simulink model "model"  (R2014a)
settings: Solver=FixedStepDiscrete  StartTime=0.0  StopTime=10.0  RelTol=1e-3
undefined symbols (not defined in the file): ECU565, motohawk_build_version, motohawk_trunc_name, motohawk_vardec_path
libraries: MotoHawk_lib x21
settings Model: MotoHawkModelGUID=11A61F78-2EA3-404C-BC5C-7D2024A9F3B7  MotoHawkModelOpenTime=2016 1 25 15 27 48.637  MotoHawkBuildVersion=007  MotoHawkBuildStats=struct('TotalFLASH',{0},'TotalEEPROM',{0},'TotalRAM',{0},'AppFLASH',{0},'AppEEPROM',{0},'AppRAM',{0},'HeapRAM',{0},'BuildSuccessCount',{7},'BuildErrorCount',{0})  MotoHawkBuildDirectory=H:\EE 5750 Lab\Lab 1\model_Build  MotoHawkBuildInfo=struct('model_name',{'model'},'motohawk_version',{'2014a_sp3.1030'},'motohawk_component_version',{'0.0.8'},'matlab_version',{'8.3.0'},'build_version',{'006'},'module_type',{'ECU565-128'},'layout_type',{'DEV'},'processor_family',{'PPC'},'processor_type',{'MPC565'},'toolchain_vendor',{'gcc-powerpc-eabi'},'toolchain_version',{'4.6.0'},'component',{0},'archive_file',{'PCM128.a'},'enable_build',{1},'fptype',{0},'flash_size',{1048576},'ee_size',{8192},'ram_size',{36864},'decram_size',{4096},'eri_table0_rev',{9},'max_eri_table_size',{65535},'fgnd_base_period_ms',{5},'bgnd_base_period_ms',{50},'build_dir',{'H:\EE 5750 Lab\Lab 1\model_Build'},'dll_name',{'model_006'},'srz_name',{'model_006'},'fgnd_stack_size',{3072},'fgnd_angle_stack_size',{0},'bgnd_stack_size',{2048},'idle_stack_size',{1024},'irq_stack_size',{1536},'heap_size',{4096},'heap_margin',{409},'install_dll_dir',{'C:\ECUFiles\TDBDLL'},'install_srz_dir',{'C:\ECUFiles\Programs'},'app_int_stack_size',{1024},'shutdown_stack_size',{1024},'mingw_dir',{'C:\Program Files (x86)\Woodward\DevelopmentTools\Toolchains\GCC\win32-pe\4_7_0'},'motohawk_dir',{'C:\Program Files (x86)\Woodward\MCS\MotoHawk\2014a_sp3.1030'},'toolchain_dir',{'C:\Program Files (x86)\Woodward\DevelopmentTools\Toolchains\GCC\powerpc-eabi\4_6_0'},'matlab_root',{'C:\Program Files\MATLAB\2014a'},'model_guid',{'11A61F78-2EA3-404C-BC5C-7D2024A9F3B7'},'build_guid',{'7B202DAE-6419-4B4F-BE95-2BA6D031F5CC'},'token_guid',{'FCE0CA5DFB76074BA85E27C6355608D2'})  MotoHawkModelSavedName=model  MotoHawkModelElapsedTime=23442.054  MotoHawkBuildGUID=7B202DAE-6419-4B4F-BE95-2BA6D031F5CC  Creator=lbaruah  LastModifiedBy=lbaruah
settings ConfigSet: Description="This Simulink Configuration Set is preconfigured  for the MotoHawk target \"ECU565-128\"."
settings OptimizationCC: InlineParams=on  InlineInvariantSignals=on  EnhancedBackFolding=on  InitFltsAndDblsToZero=on  NoFixptDivByZeroProtection=on  EfficientFloat2IntCast=on  OptimizeModelRefInitCode=on  LifeSpan=1
settings DebuggingCC: UnderspecifiedInitializationDetection=Classic  SolverPrmCheckMsg=none  InheritedTsInSrcMsg=none  TasksWithSamePriorityMsg=none
settings HardwareCC: ProdLargestAtomicInteger=Integer  ProdLargestAtomicFloat=Float  ProdEndianess=BigEndian  ProdHWDeviceType=Specified
settings ModelReferenceCC: UpdateModelReferenceTargets=AssumeUpToDate  CheckModelReferenceTargetMessage=none  ModelReferenceNumInstancesAllowed=Zero
settings RTWCC: SystemTargetFile=motohawk_ert_rtw.tlc  MakeCommand=motohawk_make_rtw  TemplateMakefile=motohawk_ert_rtw.tmf  Description=MotoHawk(tm) Rapid Prototyping  ProcessScript=motohawk_ert_rtw_make_rtw_hook
settings CodeAppCC: IgnoreCustomStorageClasses=off  MaxIdLength=100  CustomSymbolStrType=$N$R$M  CustomSymbolStrField=$H$N$M  InternalIdentifier=Classic
settings STFCustomTargetCC: ERTMultiwordTypeDef=User defined  ModelReferenceCompliant=off  ConcurrentExecutionCompliant=off  IncludeMdlTerminateFcn=off  CombineOutputUpdateFcns=on  SuppressErrorStatus=on  ERTCustomFileBanners=on  SupportContinuousTime=off  SupportNonInlinedSFcns=off  MATLABClassNameForMDSCustomization=Simulink.SoftwareTarget.ERTCustomization  GRTInterface=off  SystemTargetFile=motohawk_ert_rtw.tlc
settings ERTTargetCC: ERTMultiwordTypeDef=User defined  ERTMultiwordLength=0  GenerateSampleERTMain=off  ModelReferenceCompliant=off  IncludeMdlTerminateFcn=off  GeneratePreprocessorConditionals=Disable all  SuppressErrorStatus=on  ERTCustomFileTemplate=example_file_process.tlc

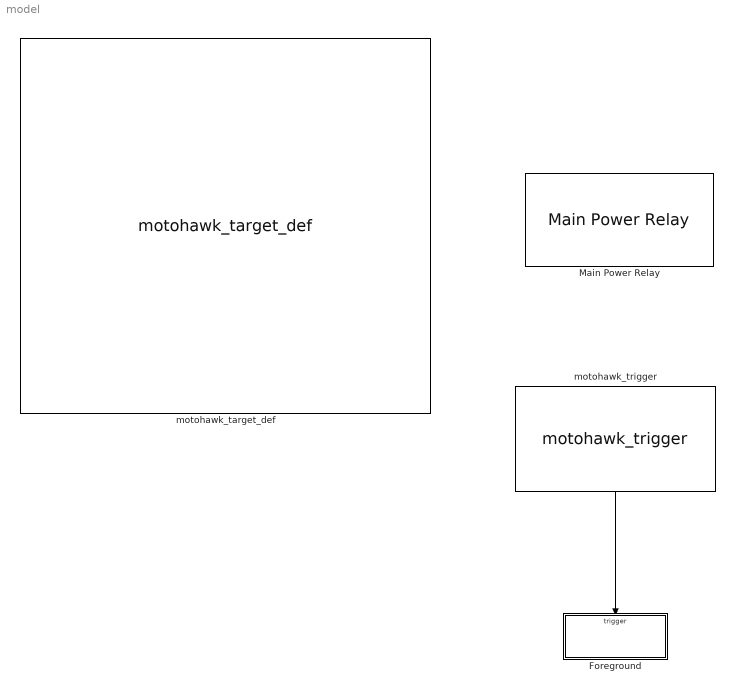
== system model ==
  Foreground : Subsystem  TreatAsAtomicUnit=on
  Main Power Relay : MotoHawk_lib/Extra Development Blocks/Main Power Relay  on_delay_count=2  off_delay_count=5  ecup_threshold=100  group='System | Main Power Relay'
  motohawk_target_def : MotoHawk_lib/motohawk_target_def  Priority=-65535  target=ECU565-128  layout=DEV  fptype=single (32 bits)  fgnd_stack_size=3*1024  fgnd_angle_stack_size=0  bgnd_stack_size=2*1024  idle_stack_size=1024  irq_stack_size=1536  app_int_stack_size=1024  shutdown_stack_size=1024  heap_size=4*1024  show_margins=off  fgnd_stack_margin=(3*1024) * 0.1  fgnd_angle_stack_margin=0  bgnd_stack_margin=(2*1024) * 0.1  idle_stack_margin=(1024) * 0.1  irq_stack_margin=(1536) * 0.1  app_int_stack_margin=(1024) * 0.1  shutdown_stack_margin=(1024) * 0.1  heap_margin=(4*1024) * 0.1  comp_name=bdroot  comp_img='KVASER_CAN_USB.jpg'  comp_security=No Encryption  comp_build_pass='mhbuild'  comp_sim_pass='mhsim'  comp_multi=off  show_filenames=off  dll_name=motohawk_trunc_name(bdroot, ['_' motohawk_build_version], 13)  srz_name=motohawk_trunc_name(bdroot, ['_' motohawk_build_version], 50)  build_dir='.'  comp_dir='.'
  motohawk_trigger : MotoHawk_lib/Trigger Blocks/motohawk_trigger  Tag=Trigger  Priority=0  trig_name=[]  trigger=FGND_RTI_PERIODIC  priority_order=0  inherited=off  run_disabled=off  override_app_monitor=off  target=ECU565_128
  wires:
  motohawk_trigger/1 -> Foreground/Trigger

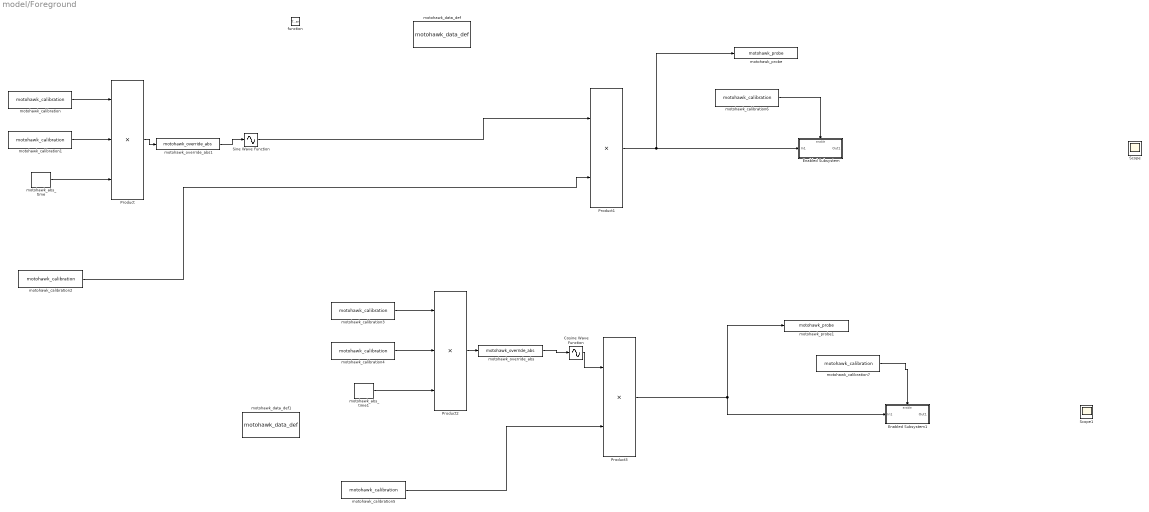
== system model/Foreground ==
  function : TriggerPort  TriggerType=function-call
  Cosine Wave Function : Sin  TimeSource=Use external signal  Phase=pi/2  SampleTime=0
  Enabled Subsystem : Subsystem  TreatAsAtomicUnit=on
  Enabled Subsystem1 : Subsystem  TreatAsAtomicUnit=on
  Product : Product  Inputs=3
  Product1 : Product
  Product2 : Product  Inputs=3
  Product3 : Product
  Scope : Scope
  Scope1 : Scope
  Sine Wave Function : Sin  TimeSource=Use external signal  SampleTime=0
  motohawk_abs_time : MotoHawk_lib/Extra Development Blocks/motohawk_abs_time  mode=Seconds (double)  width=64 bit
  motohawk_abs_time1 : MotoHawk_lib/Extra Development Blocks/motohawk_abs_time  mode=Seconds (double)  width=64 bit
  motohawk_calibration : MotoHawk_lib/Calibration & Probing Blocks/motohawk_calibration  nam='TwoPi'  val=6.28318  storage=Calibration  show_more=off  name_source=Use Parameter  data_type=Inherit from 'Default Value'  read_level=1  write_level=1  ovr_cals=on  view_as=Number  enum_struct={'Disabled', 'Enabled'}  vector_style=Wide Row  use_help_units=off  help=''  units=''  use_header_enum=off  row_header_enum={}  col_header_enum={}  use_min_max=off  min_val=-inf  max_val=inf  use_precision=off  precision=''  gain=1  offset=0  exp=1  use_mototune_group=off  mototune_group=motohawk_vardec_path(gcb)  data_stores=motohawk_sfun_calibration_data_stores
  motohawk_calibration1 : MotoHawk_lib/Calibration & Probing Blocks/motohawk_calibration  nam='f'  val=1  storage=Calibration  show_more=off  name_source=Use Parameter  data_type=Inherit from 'Default Value'  read_level=1  write_level=1  ovr_cals=on  view_as=Number  enum_struct={'Disabled', 'Enabled'}  vector_style=Wide Row  use_help_units=off  help=''  units=''  use_header_enum=off  row_header_enum={}  col_header_enum={}  use_min_max=off  min_val=-inf  max_val=inf  use_precision=off  precision=''  gain=1  offset=0  exp=1  use_mototune_group=off  mototune_group=motohawk_vardec_path(gcb)  data_stores=motohawk_sfun_calibration_data_stores
  motohawk_calibration2 : MotoHawk_lib/Calibration & Probing Blocks/motohawk_calibration  nam='Amplitude'  val=10  storage=Calibration  show_more=off  name_source=Use Parameter  data_type=Inherit from 'Default Value'  read_level=1  write_level=1  ovr_cals=on  view_as=Number  enum_struct={'Disabled', 'Enabled'}  vector_style=Wide Row  use_help_units=off  help=''  units=''  use_header_enum=off  row_header_enum={}  col_header_enum={}  use_min_max=off  min_val=-inf  max_val=inf  use_precision=off  precision=''  gain=1  offset=0  exp=1  use_mototune_group=off  mototune_group=motohawk_vardec_path(gcb)  data_stores=motohawk_sfun_calibration_data_stores
  motohawk_calibration3 : MotoHawk_lib/Calibration & Probing Blocks/motohawk_calibration  nam='TwoPi1'  val=6.28318  storage=Calibration  show_more=off  name_source=Use Parameter  data_type=Inherit from 'Default Value'  read_level=1  write_level=1  ovr_cals=on  view_as=Number  enum_struct={'Disabled', 'Enabled'}  vector_style=Wide Row  use_help_units=off  help=''  units=''  use_header_enum=off  row_header_enum={}  col_header_enum={}  use_min_max=off  min_val=-inf  max_val=inf  use_precision=off  precision=''  gain=1  offset=0  exp=1  use_mototune_group=off  mototune_group=motohawk_vardec_path(gcb)  data_stores=motohawk_sfun_calibration_data_stores
  motohawk_calibration4 : MotoHawk_lib/Calibration & Probing Blocks/motohawk_calibration  nam='f1'  val=1  storage=Calibration  show_more=off  name_source=Use Parameter  data_type=Inherit from 'Default Value'  read_level=1  write_level=1  ovr_cals=on  view_as=Number  enum_struct={'Disabled', 'Enabled'}  vector_style=Wide Row  use_help_units=off  help=''  units=''  use_header_enum=off  row_header_enum={}  col_header_enum={}  use_min_max=off  min_val=-inf  max_val=inf  use_precision=off  precision=''  gain=1  offset=0  exp=1  use_mototune_group=off  mototune_group=motohawk_vardec_path(gcb)  data_stores=motohawk_sfun_calibration_data_stores
  motohawk_calibration5 : MotoHawk_lib/Calibration & Probing Blocks/motohawk_calibration  nam='Amplitude1'  val=10  storage=Calibration  show_more=off  name_source=Use Parameter  data_type=Inherit from 'Default Value'  read_level=1  write_level=1  ovr_cals=on  view_as=Number  enum_struct={'Disabled', 'Enabled'}  vector_style=Wide Row  use_help_units=off  help=''  units=''  use_header_enum=off  row_header_enum={}  col_header_enum={}  use_min_max=off  min_val=-inf  max_val=inf  use_precision=off  precision=''  gain=1  offset=0  exp=1  use_mototune_group=off  mototune_group=motohawk_vardec_path(gcb)  data_stores=motohawk_sfun_calibration_data_stores
  motohawk_calibration6 : MotoHawk_lib/Calibration & Probing Blocks/motohawk_calibration  nam='log'  val=0  storage=Calibration  show_more=off  name_source=Use Parameter  data_type=Inherit from 'Default Value'  read_level=1  write_level=1  ovr_cals=on  view_as=Number  enum_struct={'Disabled', 'Enabled'}  vector_style=Wide Row  use_help_units=off  help=''  units=''  use_header_enum=off  row_header_enum={}  col_header_enum={}  use_min_max=off  min_val=-inf  max_val=inf  use_precision=off  precision=''  gain=1  offset=0  exp=1  use_mototune_group=off  mototune_group=motohawk_vardec_path(gcb)  data_stores=motohawk_sfun_calibration_data_stores
  motohawk_calibration7 : MotoHawk_lib/Calibration & Probing Blocks/motohawk_calibration  nam='log1'  val=0  storage=Calibration  show_more=off  name_source=Use Parameter  data_type=Inherit from 'Default Value'  read_level=1  write_level=1  ovr_cals=on  view_as=Number  enum_struct={'Disabled', 'Enabled'}  vector_style=Wide Row  use_help_units=off  help=''  units=''  use_header_enum=off  row_header_enum={}  col_header_enum={}  use_min_max=off  min_val=-inf  max_val=inf  use_precision=off  precision=''  gain=1  offset=0  exp=1  use_mototune_group=off  mototune_group=motohawk_vardec_path(gcb)  data_stores=motohawk_sfun_calibration_data_stores
  motohawk_data_def : MotoHawk_lib/Data Storage Blocks/motohawk_data_def  nam='SineData'  container_nam=''  data=zeros(1,200)  typ=double  struct_nam='MyStruct'  storage=NonVolatile  outputRef=off  use_vardec=on  window=Display  read_level=1  write_level=1  ovr_cals=on  view_as=Number  enum_struct={'Disabled', 'Enabled'}  vector_style=Wide Row  use_help_units=off  help=''  units=''  use_header_enum=off  row_header_enum=''  col_header_enum=''  use_min_max=off  min_val=-inf  max_val=inf  use_precision=off  precision=''  gain=1  offset=0  exp=1  use_mototune_group=off  mototune_group=motohawk_vardec_path(gcb)  eval_name=MyData  data_stores=motohawk_sfun_data_def_data_stores  struct_instances=motohawk_sfun_data_def_struct_instances  vardecs=motohawk_sfun_data_def_vardecs
  motohawk_data_def1 : MotoHawk_lib/Data Storage Blocks/motohawk_data_def  nam='CosineData'  container_nam=''  data=zeros(1,200)  typ=double  struct_nam='MyStruct'  storage=NonVolatile  outputRef=off  use_vardec=on  window=Display  read_level=1  write_level=1  ovr_cals=on  view_as=Number  enum_struct={'Disabled', 'Enabled'}  vector_style=Wide Row  use_help_units=off  help=''  units=''  use_header_enum=off  row_header_enum=''  col_header_enum=''  use_min_max=off  min_val=-inf  max_val=inf  use_precision=off  precision=''  gain=1  offset=0  exp=1  use_mototune_group=off  mototune_group=motohawk_vardec_path(gcb)  eval_name=MyData  data_stores=motohawk_sfun_data_def_data_stores  struct_instances=motohawk_sfun_data_def_struct_instances  vardecs=motohawk_sfun_data_def_vardecs
  motohawk_override_abs : MotoHawk_lib/Calibration & Probing Blocks/motohawk_override_abs  parent_name='Angle_Override1'  parent_val=0  show_more=off  name_source=Use Parameter  parent_read_level=1  parent_override_level=1  view_as=Number  enum_struct={'Disabled', 'Enabled'}  use_help_units=off  parent_help=''  parent_units=''  use_min_max=off  parent_min=-inf  parent_max=inf  use_precision=off  parent_precision=''  parent_gain=1  parent_offset=0  parent_exp=1  use_mototune_group=off  parent_group=motohawk_vardec_path(gcb)
  motohawk_override_abs1 : MotoHawk_lib/Calibration & Probing Blocks/motohawk_override_abs  parent_name='Angle_Override'  parent_val=0  show_more=off  name_source=Use Parameter  parent_read_level=1  parent_override_level=1  view_as=Number  enum_struct={'Disabled', 'Enabled'}  use_help_units=off  parent_help=''  parent_units=''  use_min_max=off  parent_min=-inf  parent_max=inf  use_precision=off  parent_precision=''  parent_gain=1  parent_offset=0  parent_exp=1  use_mototune_group=off  parent_group=motohawk_vardec_path(gcb)
  motohawk_probe : MotoHawk_lib/Calibration & Probing Blocks/motohawk_probe  nam='sine'  show_more=off  name_source=Use Parameter  read_level=1  view_as=Number  enum_struct={'Disabled', 'Enabled'}  vector_style=Wide Row  use_help_units=off  help=''  units=''  use_header_enum=off  row_header_enum={}  col_header_enum={}  use_min_max=off  min_val=-inf  max_val=inf  use_precision=off  precision=''  gain=1  offset=0  exp=1  use_mototune_group=off  mototune_group=motohawk_vardec_path(gcb)
  motohawk_probe1 : MotoHawk_lib/Calibration & Probing Blocks/motohawk_probe  nam='Cosine'  show_more=off  name_source=Use Parameter  read_level=1  view_as=Number  enum_struct={'Disabled', 'Enabled'}  vector_style=Wide Row  use_help_units=off  help=''  units=''  use_header_enum=off  row_header_enum={}  col_header_enum={}  use_min_max=off  min_val=-inf  max_val=inf  use_precision=off  precision=''  gain=1  offset=0  exp=1  use_mototune_group=off  mototune_group=motohawk_vardec_path(gcb)
  wires:
  motohawk_calibration/1 -> Product/1
  motohawk_calibration1/1 -> Product/2
  motohawk_abs_time/1 -> Product/3
  Sine Wave Function/1 -> Product1/1
  Product1/1 -> Enabled Subsystem/1(In1), motohawk_probe/1
  motohawk_calibration2/1 -> Product1/2
  motohawk_calibration3/1 -> Product2/1
  motohawk_calibration4/1 -> Product2/2
  motohawk_abs_time1/1 -> Product2/3
  Product3/1 -> motohawk_probe1/1, Enabled Subsystem1/1(In1)
  motohawk_calibration5/1 -> Product3/2
  Cosine Wave Function/1 -> Product3/1
  Product/1 -> motohawk_override_abs1/1
  motohawk_override_abs1/1 -> Sine Wave Function/1
  Product2/1 -> motohawk_override_abs/1
  motohawk_override_abs/1 -> Cosine Wave Function/1
  motohawk_calibration6/1 -> Enabled Subsystem/Enable
  motohawk_calibration7/1 -> Enabled Subsystem1/Enable

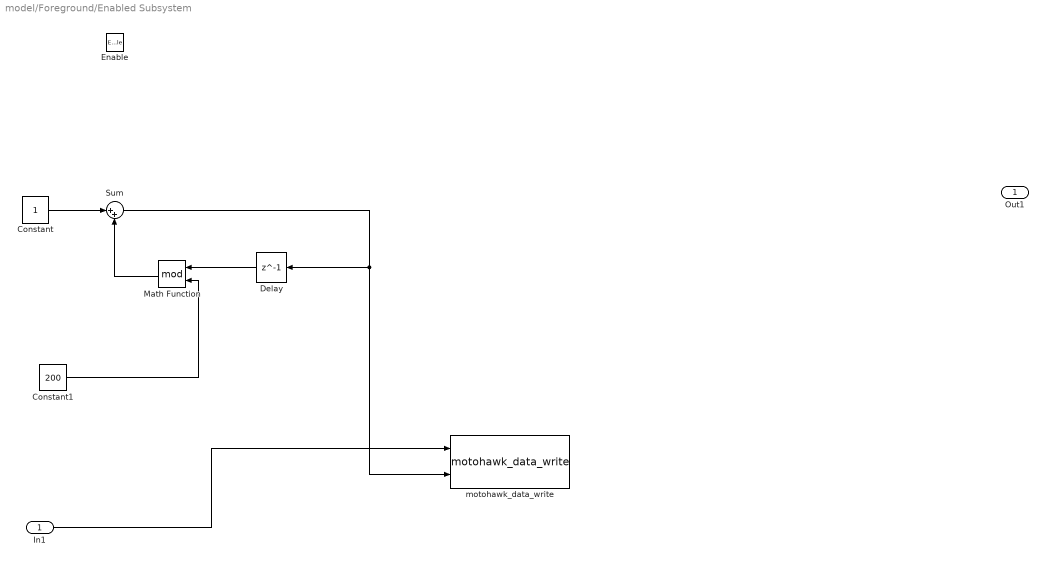
== system model/Foreground/Enabled Subsystem ==
  In1 : Inport
  Enable : EnablePort
  Constant : Constant
  Constant1 : Constant  Value=200
  Delay : Delay  DelayLength=1  InitialCondition=0
  Math Function : Math  Operator=mod  SaturateOnIntegerOverflow=on
  Sum : Sum  Inputs=|++
  motohawk_data_write : MotoHawk_lib/Data Storage Blocks/motohawk_data_write  source=Lookup By Name  structure=Vector  operation=Write scalar into location by index  sz_vec=400  sz_row=2  sz_col=9  typ=double  nam='SineData'  checkNull=on  write_read_only=off  struct_inst_name=''  struct_name='MyStruct'
  Out1 : Outport
  wires:
  Constant/1 -> Sum/1
  Math Function/1 -> Sum/2
  Constant1/1 -> Math Function/2
  Delay/1 -> Math Function/1
  Sum/1 -> Delay/1, motohawk_data_write/2
  In1/1 -> motohawk_data_write/1

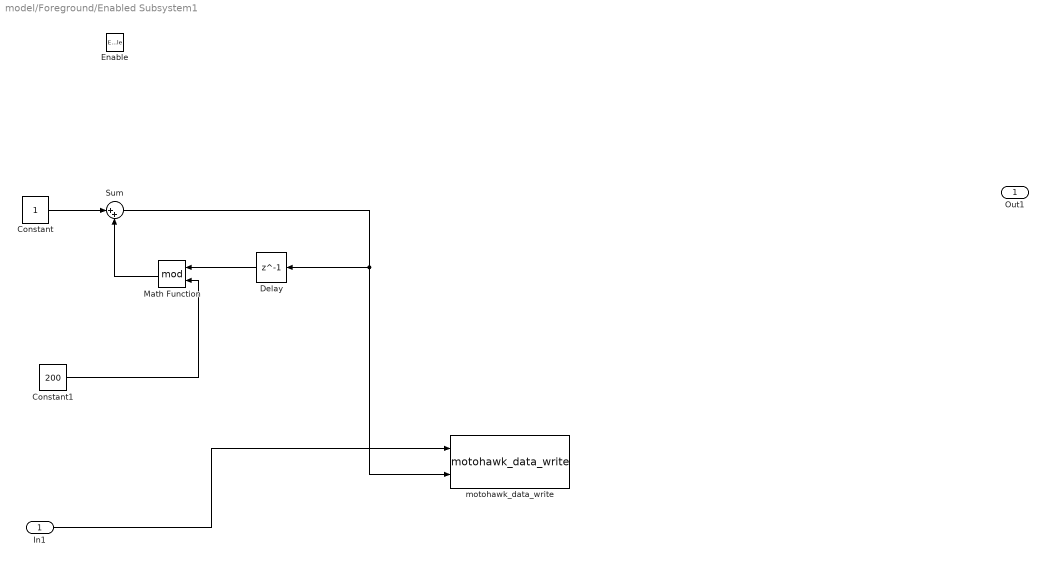
== system model/Foreground/Enabled Subsystem1 ==
  In1 : Inport
  Enable : EnablePort
  Constant : Constant
  Constant1 : Constant  Value=200
  Delay : Delay  DelayLength=1  InitialCondition=0
  Math Function : Math  Operator=mod  SaturateOnIntegerOverflow=on
  Sum : Sum  Inputs=|++
  motohawk_data_write : MotoHawk_lib/Data Storage Blocks/motohawk_data_write  source=Lookup By Name  structure=Vector  operation=Write scalar into location by index  sz_vec=400  sz_row=2  sz_col=9  typ=double  nam='CosineData'  checkNull=on  write_read_only=off  struct_inst_name=''  struct_name='MyStruct'
  Out1 : Outport
  wires:
  Constant/1 -> Sum/1
  Math Function/1 -> Sum/2
  Constant1/1 -> Math Function/2
  Delay/1 -> Math Function/1
  Sum/1 -> Delay/1, motohawk_data_write/2
  In1/1 -> motohawk_data_write/1
